simulink model "spl_smash_sd_ustf_Zdomain"  (R2022a)
settings: Solver=VariableStepDiscrete  StartTime=0.0  StopTime=0.01  RelTol=1e-3  EnableMultiTasking=on
model workspace (MAT data in the model file):
  fin = 10
values from neighbouring files (symbols this model uses):
  Ain = 1    [spl_modelparameters.m]
  ts = 1/sdm_rate    (= 1.62760416667e-07)    [spl_modelparameters.m]
  ts_audio = 1/adc_rate    (= 2.60416666667e-06)    [spl_modelparameters.m]
libraries: dspfdesign x1
settings Model: Creator=mohammed  LastModifiedBy=mohammed
settings SolverCC: AlgebraicLoopSolver=TrustRegion
settings DataIOCC: LimitDataPoints=on  SaveFormat=Array  SignalLoggingSaveFormat=ModelDataLogs  ReturnWorkspaceOutputs=off
settings OptimizationCC: InitFltsAndDblsToZero=on  LifeSpan=inf
settings DebuggingCC: SaveWithParameterizedLinksMsg=none  UnderspecifiedInitializationDetection=Classic  MergeDetectMultiDrivingBlocksExec=none  SignalResolutionControl=TryResolveAllWithWarning  SolverPrmCheckMsg=warning  MultiTaskDSMMsg=warning  MultiTaskCondExecSysMsg=none  FcnCallInpInsideContextMsg=warning  UnconnectedInputMsg=warning  UnconnectedOutputMsg=warning  UnconnectedLineMsg=warning  SFUnexpectedBacktrackingDiag=warning  SFNoUnconditionalDefaultTransitionDiag=warning  SFExecutionAtInitializationDiag=none  SFMachineParentedDataDiag=warning  ArithmeticOperatorsInVariantConditions=warning
settings HardwareCC: ProdBitPerPointer=32  ProdBitPerSizeT=32  ProdBitPerPtrDiffT=32  ProdLargestAtomicFloat=None  ProdIntDivRoundTo=Undefined  ProdEndianess=Unspecified  ProdWordSize=32  ProdHWDeviceType=32-bit Generic
settings ModelReferenceCC: PropagateSignalLabelsOutOfModel=off
settings CodeAppCC: StateflowObjectComments=on
settings GRTTargetCC: TargetFcnLib=ansi_tfl_tmw.mat  TargetLangStandard=C89/C90 (ANSI)  CombineOutputUpdateFcns=off  GRTInterface=on
settings ConfigComp: CovMetricSettings=dw  CovSaveCumulativeToWorkspaceVar=on  CovSaveSingleToWorkspaceVar=on

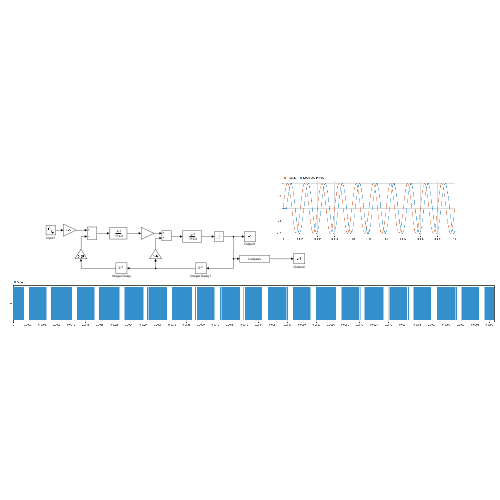
[thumbnail: Simulink's stored preview of the top-level diagram]
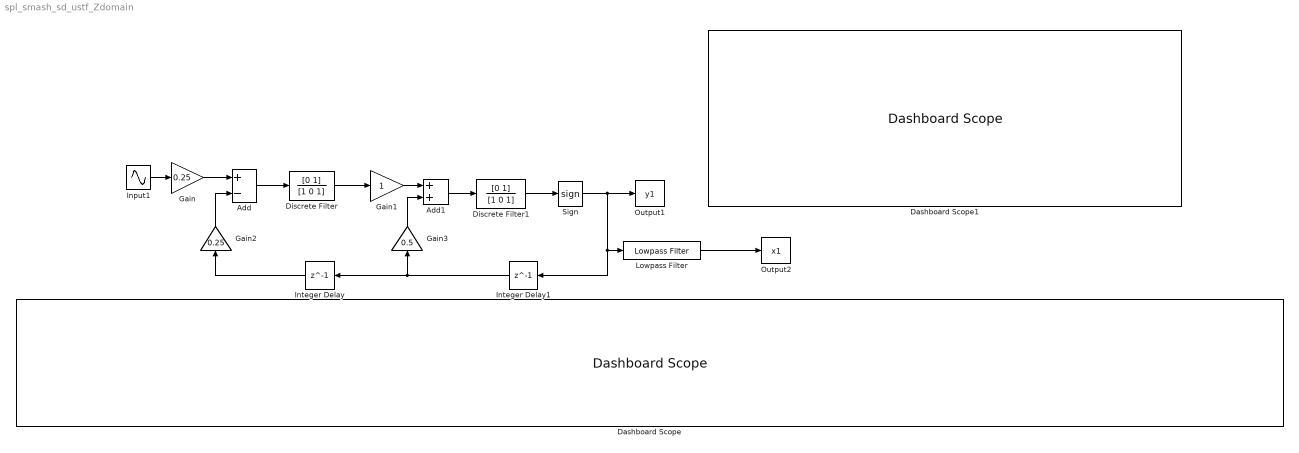
== system spl_smash_sd_ustf_Zdomain ==
  Add : Sum  Inputs=+-
  Add1 : Sum
  Dashboard Scope : DashboardScope
  Dashboard Scope1 : DashboardScope
  Discrete Filter : DiscreteFilter  Numerator=[0 1]  Denominator=[1 0 1]  SampleTime=ts
  Discrete Filter1 : DiscreteFilter  Numerator=[0 1]  Denominator=[1 0 1]  SampleTime=ts
  Gain : Gain  Gain=0.25
  Gain1 : Gain
  Gain2 : Gain  Gain=0.25
  Gain3 : Gain  Gain=0.5
  Input1 : Sin  Amplitude=Ain  Frequency=2*pi*1000  SampleTime=ts_audio
  Integer Delay : Delay  DelayLength=1  SampleTime=ts
  Integer Delay1 : Delay  DelayLength=1  SampleTime=ts
  Lowpass Filter : dspfdesign/Lowpass Filter  FilterType=FIR  DesignForMinimumOrder=on  FilterOrder=50  PassbandFrequency=fir_freq1  StopbandFrequency=fir_freq2  PassbandRipple=0.1  StopbandAttenuation=60  InheritSampleRate=off  SampleRate=sdm_rate  SimulateUsing=Interpreted execution  roundingMode=Floor  coeffsDataTypeStr=fixdt(1,16)
  Output1 : ToWorkspace  VariableName=y1  SampleTime=ts
  Output2 : ToWorkspace  VariableName=x1  SampleTime=ts
  Sign : Signum
  wires:
  Gain/1 -> Add/1
  Add/1 -> Discrete Filter/1
  Gain1/1 -> Add1/1
  Add1/1 -> Discrete Filter1/1
  Discrete Filter/1 -> Gain1/1
  Gain2/1 -> Add/2
  Gain3/1 -> Add1/2
  Discrete Filter1/1 -> Sign/1
  Input1/1 -> Gain/1
  Sign/1 -> Output1/1, Lowpass Filter/1, Integer Delay1/1
  Lowpass Filter/1 -> Output2/1
  Integer Delay/1 -> Gain2/1
  Integer Delay1/1 -> Integer Delay/1, Gain3/1
